simulink model "model_6_block_pipeline"  (R2026a)
settings: Solver=VariableStepAuto  StopTime=100
undefined symbols (not defined in the file): m, n
settings Model: Creator=Nilesh Banik  LastModifiedBy=Nilesh Banik

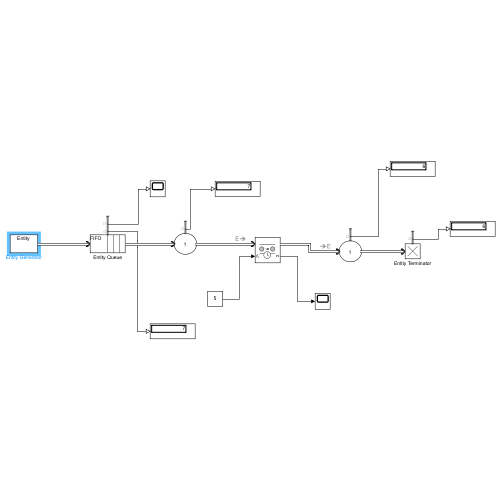
[thumbnail: Simulink's stored preview of the top-level diagram]
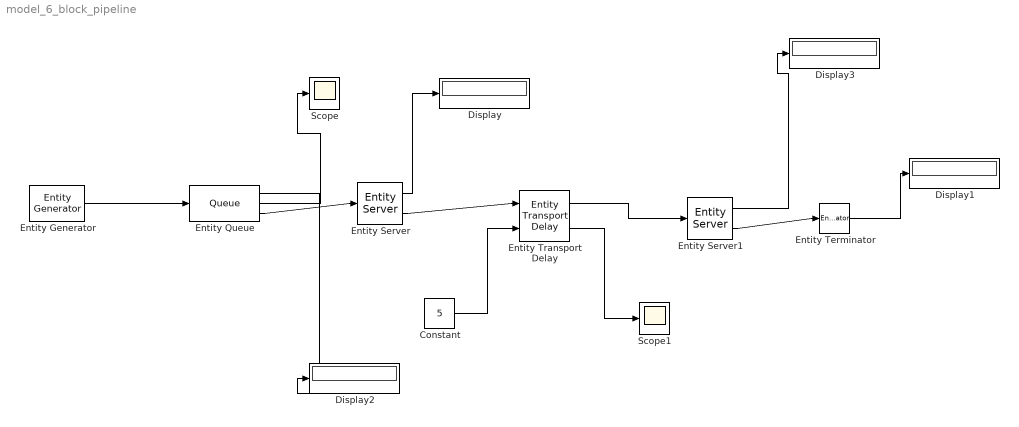
== system model_6_block_pipeline ==
  Constant : Constant  Value=5
  Display{,1..3} (4 alike) : Display
  Entity Transport Delay : EntityTransportDelay  InputPortMessageModes=m,n  OutputPortMessageModes=m,n  ShowNumberEntitiesInBlock=on
  Entity Generator : EntityGenerator  OutputPortMessageModes=m  Period=15  EntityType=Structured  EntityTypeName=Entity
  Entity Queue : Queue  InputPortMessageModes=m  OutputPortMessageModes=n,n,m  Capacity=10  NumberEntitiesDeparted=on  NumberEntitiesInBlock=on
      settings: OutputPortMap=o0,o1,o5
  Entity Server : EntityServer  InputPortMessageModes=m  OutputPortMessageModes=n,m  Capacity=1  ServiceTimeValue=10  NumberEntitiesDeparted=on
      settings: OutputPortMap=o0,o9
  Entity Server1 : EntityServer  InputPortMessageModes=m  OutputPortMessageModes=n,m  Capacity=1  ServiceTimeValue=8  NumberEntitiesDeparted=on
      settings: OutputPortMap=o0,o9
  Entity Terminator : EntityTerminator  InputPortMessageModes=m  NumberEntitiesArrived=on
      settings: OutputPortMap=o0
  Scope : Scope
      settings: ActiveDisplayYMinimum=-0.7251537001794679  ActiveDisplayYMaximum=2.0034395352979537
  Scope1 : Scope
      settings: ActiveDisplayYMinimum=-0.32485258304328091  ActiveDisplayYMaximum=1.2704993700817198
  wires:
  Entity Generator/1 -> Entity Queue/1
  Entity Queue/3 -> Entity Server/1
  Entity Server/2 -> Entity Transport Delay/1
  Entity Transport Delay/1 -> Entity Server1/1
  Entity Server1/2 -> Entity Terminator/1
  Constant/1 -> Entity Transport Delay/2
  Entity Queue/2 -> Scope/1
  Entity Transport Delay/2 -> Scope1/1
  Entity Server/1 -> Display/1
  Entity Terminator/1 -> Display1/1
  Entity Queue/1 -> Display2/1
  Entity Server1/1 -> Display3/1
